simulink model "ControlledGrid"  (R2015b)
settings: configuration reference "ControlConfig" (kept outside this file)
InitFcn:
  | ControlInit();
undefined symbols (not defined in the file or in its folder): D1, Delta, Fnom, Grid_F, Grid_V, Rad2Deg, Ts
libraries: powerlib x16, powerlib_meascontrol x4, simulink x1
settings Model: Creator=Emilio  LastModifiedBy=Emilio
settings ConfigSetRef: SourceLocation=Base Workspace

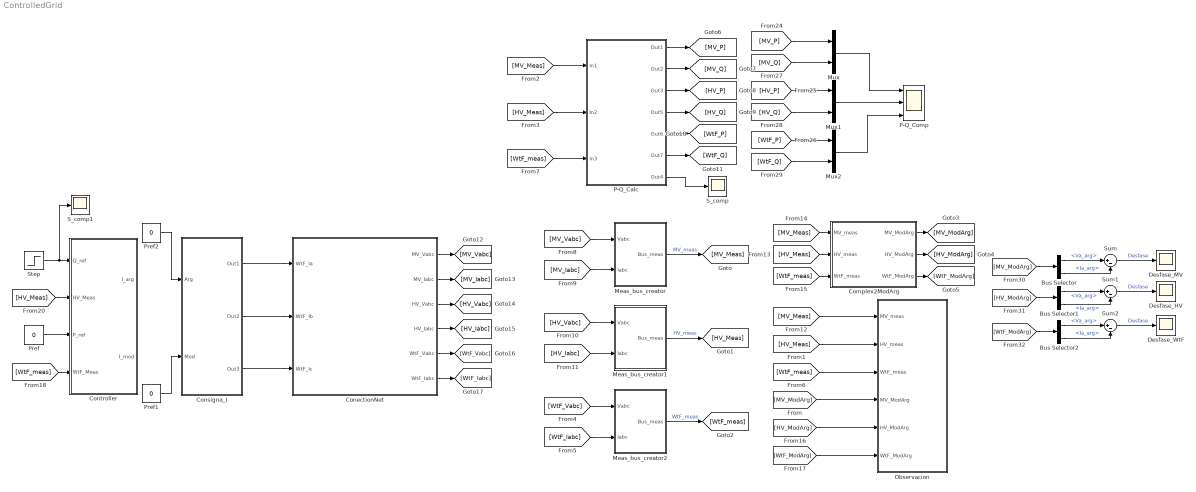
== system ControlledGrid ==
  Bus Selector : BusSelector  OutputSignals=V_ModArg.Va_arg,I_ModArg.Ia_arg
  Bus Selector1 : BusSelector  OutputSignals=V_ModArg.Va_arg,I_ModArg.Ia_arg
  Bus Selector2 : BusSelector  OutputSignals=V_ModArg.Va_arg,I_ModArg.Ia_arg
  Complex2ModArg : Subsystem
  ConectionNet : Subsystem
  Consigna_I : Subsystem
  Controller : Subsystem
  Desfase_HV : Scope
  Desfase_MV : Scope
  Desfase_WtF : Scope
  Meas_bus_creator : Subsystem
  Meas_bus_creator1 : Subsystem
  Meas_bus_creator2 : Subsystem
  Mux : Mux  Inputs=2
  Mux1 : Mux  Inputs=2
  Mux2 : Mux  Inputs=2
  Observacion : Subsystem
  P-Q_Calc : Subsystem
  P-Q_Comp : Scope  NumInputPorts=3
  Pref : Constant  Value=0
  Pref1 : Constant  Value=0
  Pref2 : Constant  Value=0
  S_comp : Scope
  S_comp1 : Scope
  Step : Step  After=4e6  SampleTime=0
  Sum : Sum  Inputs=|+-
  Sum1 : Sum  Inputs=|+-
  Sum2 : Sum  Inputs=|+-
  wires:
  [MV_Meas] -> P-Q_Calc/1(In1)
  [HV_Meas] -> P-Q_Calc/2(In2)
  P-Q_Calc/7(Out4) -> S_comp/1
  [MV_Vabc] -> Meas_bus_creator/1(Vabc)
  [MV_Iabc] -> Meas_bus_creator/2(Iabc)
  Meas_bus_creator/1(Bus_meas) -> [MV_Meas]  "MV_meas"
  [HV_Vabc] -> Meas_bus_creator1/1(Vabc)
  [HV_Iabc] -> Meas_bus_creator1/2(Iabc)
  Meas_bus_creator1/1(Bus_meas) -> [HV_Meas]  "HV_meas"
  [WtF_Vabc] -> Meas_bus_creator2/1(Vabc)
  [WtF_Iabc] -> Meas_bus_creator2/2(Iabc)
  Meas_bus_creator2/1(Bus_meas) -> [WtF_meas]  "WtF_meas"
  [WtF_meas] -> P-Q_Calc/3(In3)
  [MV_Meas] -> Observacion/1(MV_meas)
  [HV_Meas] -> Observacion/2(HV_meas)
  [WtF_meas] -> Observacion/3(WtF_meas)
  [MV_ModArg] -> Observacion/4(MV_ModArg)
  [HV_ModArg] -> Observacion/5(HV_ModArg)
  [WtF_ModArg] -> Observacion/6(WtF_ModArg)
  P-Q_Calc/1(Out1) -> [MV_P]
  P-Q_Calc/2(Out2) -> [MV_Q]
  P-Q_Calc/3(Out3) -> [HV_P]
  P-Q_Calc/4(Out5) -> [HV_Q]
  P-Q_Calc/5(Out6) -> [WtF_P]
  P-Q_Calc/6(Out7) -> [WtF_Q]
  ConectionNet/1(MV_Vabc) -> [MV_Vabc]
  ConectionNet/2(MV_Iabc) -> [MV_Iabc]
  ConectionNet/3(HV_Vabc) -> [HV_Vabc]
  ConectionNet/4(HV_Iabc) -> [HV_Iabc]
  ConectionNet/5(WtF_Vabc) -> [WtF_Vabc]
  ConectionNet/6(WtF_Iabc) -> [WtF_Iabc]
  [MV_Meas] -> Complex2ModArg/1(MV_meas)
  [HV_Meas] -> Complex2ModArg/2(HV_meas)
  [WtF_meas] -> Complex2ModArg/3(WtF_meas)
  Complex2ModArg/1(MV_ModArg) -> [MV_ModArg]
  Complex2ModArg/2(HV_ModArg) -> [HV_ModArg]
  Complex2ModArg/3(WtF_ModArg) -> [WtF_ModArg]
  [MV_P] -> Mux/1
  [MV_Q] -> Mux/2
  [HV_Q] -> Mux1/2
  [HV_P] -> Mux1/1
  [WtF_P] -> Mux2/1
  [WtF_Q] -> Mux2/2
  Mux/1 -> P-Q_Comp/1
  Mux1/1 -> P-Q_Comp/2
  Mux2/1 -> P-Q_Comp/3
  [MV_ModArg] -> Bus Selector/1
  Bus Selector/1 -> Sum/1  "<Va_arg>"
  Bus Selector/2 -> Sum/2  "<Ia_arg>"
  Sum/1 -> Desfase_MV/1  "Desfase"
  [HV_ModArg] -> Bus Selector1/1
  Bus Selector1/1 -> Sum1/1  "<Va_arg>"
  Bus Selector1/2 -> Sum1/2  "<Ia_arg>"
  Sum1/1 -> Desfase_HV/1  "Desfase"
  Bus Selector2/1 -> Sum2/1  "<Va_arg>"
  Bus Selector2/2 -> Sum2/2  "<Ia_arg>"
  Sum2/1 -> Desfase_WtF/1  "Desfase"
  [WtF_ModArg] -> Bus Selector2/1
  Step/1 -> S_comp1/1, Controller/1(Q_ref)
  [HV_Meas] -> Controller/2(HV_Meas)
  Pref/1 -> Controller/3(P_ref)
  [WtF_meas] -> Controller/4(WtF_Meas)
  Consigna_I/1(Out1) -> ConectionNet/1(WtF_Ia)
  Consigna_I/2(Out2) -> ConectionNet/2(WtF_Ib)
  Consigna_I/3(Out3) -> ConectionNet/3(WtF_Ic)
  Pref1/1 -> Consigna_I/2(Mod)
  Pref2/1 -> Consigna_I/1(Arg)

== system ControlledGrid/Complex2ModArg ==
  MV_meas : Inport
  HV_meas : Inport  Port=2
  WtF_meas : Inport  Port=3
  Bus Creator1 : BusCreator  Inputs=2
  Bus Creator2 : BusCreator  Inputs=2
  Bus Creator3 : BusCreator  Inputs=2
  Bus Selector3 : BusSelector  OutputSignals=V_meas.Va,V_meas.Vb,V_meas.Vc,I_meas.Ia,I_meas.Ib,I_meas.Ic
  Bus Selector4 : BusSelector  OutputSignals=V_meas.Va,V_meas.Vb,V_meas.Vc,I_meas.Ia,I_meas.Ib,I_meas.Ic
  Bus Selector5 : BusSelector  OutputSignals=V_meas.Va,V_meas.Vb,V_meas.Vc,I_meas.Ia,I_meas.Ib,I_meas.Ic
  HV_mod&arg : Subsystem
  MV_mod&arg : Subsystem
  WtF_mod&arg : Subsystem
  MV_ModArg : Outport
  HV_ModArg : Outport  Port=2
  WtF_ModArg : Outport  Port=3
  wires:
  Bus Selector4/1 -> WtF_mod&arg/1(In1)  "<Va>"
  Bus Selector3/1 -> HV_mod&arg/1(In1)  "<Va>"
  Bus Selector3/2 -> HV_mod&arg/2(In2)  "<Vb>"
  Bus Selector3/3 -> HV_mod&arg/3(In3)  "<Vc>"
  Bus Selector3/4 -> HV_mod&arg/4(In4)  "<Ia>"
  Bus Selector3/6 -> HV_mod&arg/6(In6)  "<Ic>"
  HV_mod&arg/1(Out1) -> Bus Creator3/1
  HV_meas/1 -> Bus Selector3/1
  HV_mod&arg/2(Out2) -> Bus Creator3/2
  WtF_meas/1 -> Bus Selector4/1
  Bus Selector3/5 -> HV_mod&arg/5(In5)  "<Ib>"
  Bus Selector4/6 -> WtF_mod&arg/6(In6)  "<Ic>"
  MV_mod&arg/1(Out1) -> Bus Creator2/1
  Bus Selector5/3 -> MV_mod&arg/3(In3)  "<Vc>"
  Bus Selector4/3 -> WtF_mod&arg/3(In3)  "<Vc>"
  Bus Selector4/2 -> WtF_mod&arg/2(In2)  "<Vb>"
  Bus Selector4/5 -> WtF_mod&arg/5(In5)  "<Ib>"
  Bus Creator3/1 -> HV_ModArg/1  "HV_ModArg"
  Bus Selector5/1 -> MV_mod&arg/1(In1)  "<Va>"
  Bus Selector5/6 -> MV_mod&arg/6(In6)  "<Ic>"
  Bus Selector5/5 -> MV_mod&arg/5(In5)  "<Ib>"
  Bus Creator2/1 -> MV_ModArg/1  "MV_ModArg"
  Bus Selector5/2 -> MV_mod&arg/2(In2)  "<Vb>"
  Bus Creator1/1 -> WtF_ModArg/1  "WtF_ModArg"
  WtF_mod&arg/1(Out1) -> Bus Creator1/1
  WtF_mod&arg/2(Out2) -> Bus Creator1/2
  MV_mod&arg/2(Out2) -> Bus Creator2/2
  Bus Selector4/4 -> WtF_mod&arg/4(In4)  "<Ia>"
  Bus Selector5/4 -> MV_mod&arg/4(In4)  "<Ia>"
  MV_meas/1 -> Bus Selector5/1

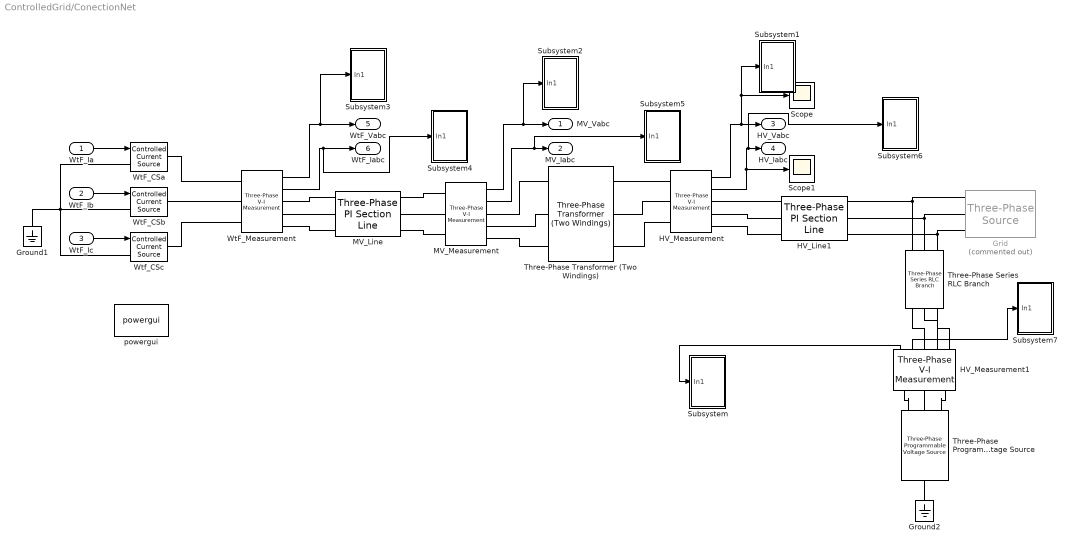
== system ControlledGrid/ConectionNet ==
  WtF_Ia : Inport
  WtF_Ib : Inport  Port=2
  WtF_Ic : Inport  Port=3
  Grid : powerlib/Electrical Sources/Three-Phase Source  Commented=on  InternalConnection=Yg  VoltagePhases=off  Voltage=Grid_V  PhaseAngle=0  Voltage_phases=[25e3 25e3 25e3]/sqrt(3)  PhaseAngles_phases=[0 -120 +120]  Frequency=Grid_F  NonIdealSource=on  SpecifyImpedance=on  Resistance=0.8929  Inductance=16.58e-3  ShortCircuitLevel=100e6  BaseVoltage=25e3  XRratio=7  BusType=PQ  Pref=10e3  Qref=0  Prefabc=[10e3, 10e3, 10e3]  Qrefabc=[0, 0, 0]  Qmin=-inf  Qmax=inf
  Ground1 : powerlib/Elements/Ground  LConnTagsString=a
  Ground2 : powerlib/Elements/Ground  LConnTagsString=a
  HV_Line1 : powerlib/Elements/Three-Phase PI Section Line  LConnTagsString=a|b|c  RConnTagsString=A|B|C  Frequency=Fnom  Resistances=[ 0.01273 0.3864]  Inductances="[ 0.9337e-3  4.1264e-3]"  Capacitances=[0.16e-6 0.16e-6]  Length=100
  HV_Measurement : powerlib/Measurements/Three-Phase V-I Measurement  VoltageMeasurement=phase-to-ground  SetLabelV=off  LabelV=HV_Vabc  Vpu=off  VpuLL=off  CurrentMeasurement=yes  SetLabelI=off  LabelI=HV_Iabc  Ipu=off  Pbase=100e6  Vbase=500e3  OutputType=Complex  PhasorSimulation=on  PSBequivalent=0
  HV_Measurement1 : powerlib/Measurements/Three-Phase V-I Measurement  VoltageMeasurement=phase-to-ground  SetLabelV=off  LabelV=HV_Vabc  Vpu=off  VpuLL=off  CurrentMeasurement=yes  SetLabelI=off  LabelI=HV_Iabc  Ipu=off  Pbase=100e6  Vbase=500e3  OutputType=Complex  PhasorSimulation=on  PSBequivalent=0
  MV_Line : powerlib/Elements/Three-Phase PI Section Line  LConnTagsString=a|b|c  RConnTagsString=A|B|C  Frequency=50  Resistances=[ 0.01273 0.3864]  Inductances="[ 0.9337e-3  4.1264e-3]"  Capacitances="[ 0.16e-6  0.16e-6]"  Length=20
  MV_Measurement : powerlib/Measurements/Three-Phase V-I Measurement  VoltageMeasurement=phase-to-ground  SetLabelV=off  LabelV=MV_Vabc  Vpu=off  VpuLL=off  CurrentMeasurement=yes  SetLabelI=off  LabelI=MV_Iabc  Ipu=off  Pbase=100e6  Vbase=500e3  OutputType=Complex  PhasorSimulation=on  PSBequivalent=0
  Scope : Scope
  Scope1 : Scope
  Subsystem : Subsystem
  Subsystem1 : Subsystem
  Subsystem2 : Subsystem
  Subsystem3 : Subsystem
  Subsystem4 : Subsystem
  Subsystem5 : Subsystem
  Subsystem6 : Subsystem
  Subsystem7 : Subsystem
  Three-Phase Programmable Voltage Source : powerlib/Electrical Sources/Three-Phase Programmable Voltage Source  PositiveSequence="[Grid_V  0 Fnom]"  VariationEntity=Amplitude  VariationType=Modulation  VariationTypeAlt=Step  VariationStep=0.5  VariationRate=10  VariationMagnitude=0  VariationFrequency=0.10  VariationTiming=[0 10]  VariationPhaseA=off  Amplitudes=[1 0.8 1.2 1.0]  TimeValues=[0 0.1 0.15 0.2]  HarmonicGeneration=off  HarmonicA=[3 0.2 -25 0]  HarmonicB=[2 0.15 35 2]  Timing="[0.05  3]"  BusType=PQ  Pref=0  Qref=0  Qmin=-inf  Qmax=inf
  Three-Phase Series RLC Branch : powerlib/Elements/Three-Phase Series RLC Branch  LConnTagsString=A|B|C  RConnTagsString=A|B|C  BranchType=RL  Resistance=1  Inductance=7  Capacitance=0  Measurements=None
  Three-Phase Transformer (Two Windings) : powerlib/Elements/Three-Phase Transformer (Two Windings)  Winding1Connection=Delta (D1)  Winding2Connection=Delta (D1)  CoreType=Three single-phase transformers  SetSaturation=off  Hysteresis=off  DataFile='hysteresis'  SetInitialFlux=off  Measurements=None  UNITS=SI  NominalPower=[ 100e3 , 50 ]  Winding1=[22000 9.68 0.030812]  Winding2=[4e+05 3200 10.186]  Rm=2.42e+06  Lm=7703.1  L0=7.7033  Saturation=[0 0;0.0089072 68.613;3.7113 86.91]  InitialFluxes=[45.742 -45.742 40.024]  MoreParameters=off  BreakLoop=off  DataType=on  TransfoNumber=1
  WtF_CSa : powerlib/Electrical Sources/Controlled Current Source  Initialize=on  Source_Type=AC  Amplitude=0  Phase=0  Frequency=Fnom  Measurements=None
  WtF_CSb : powerlib/Electrical Sources/Controlled Current Source  Initialize=on  Source_Type=AC  Amplitude=0  Phase=120  Frequency=Fnom  Measurements=None
  WtF_Measurement : powerlib/Measurements/Three-Phase V-I Measurement  VoltageMeasurement=phase-to-ground  SetLabelV=off  LabelV=WtF_Vabc  Vpu=off  VpuLL=off  CurrentMeasurement=yes  SetLabelI=off  LabelI=WtF_Iabc  Ipu=off  Pbase=100e6  Vbase=500e3  OutputType=Complex  PhasorSimulation=on  PSBequivalent=0
  Wtf_CSc : powerlib/Electrical Sources/Controlled Current Source  Initialize=on  Source_Type=AC  Amplitude=0  Phase=-120  Frequency=Fnom  Measurements=None
  powergui : powerlib/powergui  Priority=1  SimulationMode=Phasor  SolverType=Tustin/Backward Euler (TBE)  SampleTime=50e-6  frequency=Fnom  SPID=off  DisableSnubberDevices=off  DisableRonSwitches=off  DisableVfSwitches=off  SwTol=0  DisplayEquations=off  Interpol=off  ExternalGateDelay=off  methode=off  Ts=10  FunctionMessages=off  echomessages=off  HookPort=off  EnableUseOfTLC=off  x0status=blocks  frequencyindice=50  Pbase=100e6  ErrMax=1e-4  Iterations=50  UnitsV=V  UnitsW=W  buscounter=0  RestoreLinks=warning  ResistiveCurrentMeasurement=off  Frange=[0:2:500]  Ylog=off  Xlog=on  ShowGrid=off  save=off  variable=ZData  structure=0  ZoomFFT=off  StartTime=0.0  cycles=1  DisplayStyle=1  fundamental=60  FreqAxis=off  MaxFrequency=1000  frequencyindicesteady=1  RmsSteady=1  display=off
  MV_Vabc : Outport
  MV_Iabc : Outport  Port=2
  HV_Vabc : Outport  Port=3
  HV_Iabc : Outport  Port=4
  WtF_Vabc : Outport  Port=5
  WtF_Iabc : Outport  Port=6
  wires:
  WtF_Ia/1 -> WtF_CSa/1
  WtF_Ib/1 -> WtF_CSb/1
  WtF_Ic/1 -> Wtf_CSc/1
  MV_Measurement/1 -> Subsystem2/1(In1), MV_Vabc/1
  HV_Measurement/1 -> Subsystem1/1(In1), Scope/1, HV_Vabc/1
  HV_Measurement/2 -> Subsystem6/1(In1), HV_Iabc/1, Scope1/1
  MV_Measurement/2 -> Subsystem5/1(In1), MV_Iabc/1
  WtF_Measurement/1 -> Subsystem3/1(In1), WtF_Vabc/1
  WtF_Measurement/2 -> WtF_Iabc/1, Subsystem4/1(In1)
  HV_Measurement1/2 -> Subsystem7/1(In1)
  HV_Measurement1/1 -> Subsystem/1(In1)
  connections:
  HV_Measurement/LConn2 -- Three-Phase Transformer (Two Windings)/RConn2
  Three-Phase Series RLC Branch/LConn3 -- HV_Line1/RConn3 -- Grid/RConn1
  Three-Phase Series RLC Branch/LConn1 -- Grid/RConn3 -- HV_Line1/RConn1
  Three-Phase Series RLC Branch/LConn2 -- HV_Line1/RConn2 -- Grid/RConn2
  HV_Measurement/LConn1 -- Three-Phase Transformer (Two Windings)/RConn1
  HV_Measurement/LConn3 -- Three-Phase Transformer (Two Windings)/RConn3
  MV_Measurement/RConn2 -- Three-Phase Transformer (Two Windings)/LConn2
  MV_Measurement/RConn3 -- Three-Phase Transformer (Two Windings)/LConn3
  MV_Measurement/RConn1 -- Three-Phase Transformer (Two Windings)/LConn1
  MV_Line/RConn1 -- MV_Measurement/LConn1
  MV_Line/RConn3 -- MV_Measurement/LConn3
  WtF_Measurement/LConn3 -- Wtf_CSc/RConn1
  WtF_Measurement/LConn1 -- WtF_CSa/RConn1
  MV_Line/RConn2 -- MV_Measurement/LConn2
  WtF_Measurement/LConn2 -- WtF_CSb/RConn1
  WtF_Measurement/RConn3 -- MV_Line/LConn3
  WtF_Measurement/RConn2 -- MV_Line/LConn2
  WtF_Measurement/RConn1 -- MV_Line/LConn1
  Wtf_CSc/LConn1 -- Ground1/LConn1 -- WtF_CSb/LConn1 -- WtF_CSa/LConn1
  Three-Phase Programmable Voltage Source/RConn1 -- HV_Measurement1/LConn1
  Three-Phase Programmable Voltage Source/RConn2 -- HV_Measurement1/LConn2
  Three-Phase Programmable Voltage Source/RConn3 -- HV_Measurement1/LConn3
  HV_Measurement1/RConn1 -- Three-Phase Series RLC Branch/RConn1
  HV_Measurement1/RConn2 -- Three-Phase Series RLC Branch/RConn2
  HV_Measurement1/RConn3 -- Three-Phase Series RLC Branch/RConn3
  Ground2/LConn1 -- Three-Phase Programmable Voltage Source/LConn1
  HV_Line1/LConn1 -- HV_Measurement/RConn1
  HV_Measurement/RConn2 -- HV_Line1/LConn2
  HV_Measurement/RConn3 -- HV_Line1/LConn3

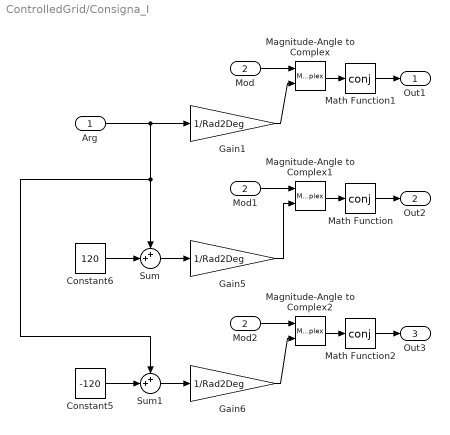
== system ControlledGrid/Consigna_I ==
  Arg : Inport
  Mod : Inport  Port=2
  Constant5 : Constant  Value=-120
  Constant6 : Constant  Value=120
  Gain1 : Gain  Gain=1/Rad2Deg
  Gain5 : Gain  Gain=1/Rad2Deg
  Gain6 : Gain  Gain=1/Rad2Deg
  Magnitude-Angle to Complex : MagnitudeAngleToComplex
  Magnitude-Angle to Complex1 : MagnitudeAngleToComplex
  Magnitude-Angle to Complex2 : MagnitudeAngleToComplex
  Math Function : Math  Operator=conj  SaturateOnIntegerOverflow=on
  Math Function1 : Math  Operator=conj  SaturateOnIntegerOverflow=on
  Math Function2 : Math  Operator=conj  SaturateOnIntegerOverflow=on
  Mod1 : InportShadow  Port=2
  Mod2 : InportShadow  Port=2
  Sum : Sum  Inputs=++|
  Sum1 : Sum  Inputs=++|
  Out1 : Outport
  Out2 : Outport  Port=2
  Out3 : Outport  Port=3
  wires:
  Gain1/1 -> Magnitude-Angle to Complex/2
  Constant6/1 -> Sum/2
  Sum/1 -> Gain5/1
  Constant5/1 -> Sum1/2
  Sum1/1 -> Gain6/1
  Arg/1 -> Sum1/1, Sum/1, Gain1/1
  Mod/1 -> Magnitude-Angle to Complex/1
  Mod1/1 -> Magnitude-Angle to Complex1/1
  Mod2/1 -> Magnitude-Angle to Complex2/1
  Gain6/1 -> Magnitude-Angle to Complex2/2
  Gain5/1 -> Magnitude-Angle to Complex1/2
  Magnitude-Angle to Complex2/1 -> Math Function2/1
  Magnitude-Angle to Complex1/1 -> Math Function/1
  Magnitude-Angle to Complex/1 -> Math Function1/1
  Math Function/1 -> Out2/1
  Math Function1/1 -> Out1/1
  Math Function2/1 -> Out3/1

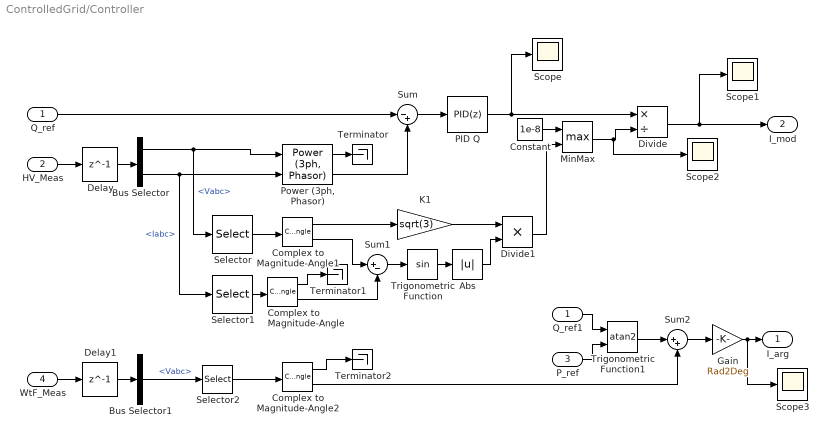
== system ControlledGrid/Controller ==
  Q_ref : Inport
  HV_Meas : Inport  Port=2  OutDataTypeStr=Bus: HV_meas
  P_ref : Inport  Port=3
  WtF_Meas : Inport  Port=4  OutDataTypeStr=Bus: WtF_meas
  Abs : Abs
  Bus Selector : BusSelector  OutputSignals=V_meas.Vabc,I_meas.Iabc
  Bus Selector1 : BusSelector  OutputSignals=V_meas.Vabc
  Complex to Magnitude-Angle : ComplexToMagnitudeAngle
  Complex to Magnitude-Angle1 : ComplexToMagnitudeAngle
  Complex to Magnitude-Angle2 : ComplexToMagnitudeAngle
  Constant : Constant  Value=1e-8
  Delay : Delay  DelayLength=1  InitialCondition=0  SampleTime=Ts
  Delay1 : Delay  DelayLength=1  InitialCondition=0  SampleTime=Ts
  Divide : Product  Inputs=*/
  Divide1 : Product  Inputs=**
  Gain : Gain  Gain=Rad2Deg
  K1 : Gain  Gain=sqrt(3)  SaturateOnIntegerOverflow=on  OutDataTypeStr=Inherit: Same as input  ParamDataTypeStr=Inherit: Same as input
  MinMax : MinMax  Function=max  Inputs=2
  PID Q : simulink/Continuous/PID Controller  Controller=PID  TimeDomain=Discrete-time  SampleTime=Ts  IntegratorMethod=Forward Euler  FilterMethod=Forward Euler  Form=Parallel  UseFilter=on  ControllerParametersSource=internal  P=1.25  I=0  D=0  N=100  InitialConditionSource=internal  InitialConditionForIntegrator=0  InitialConditionForFilter=0  ExternalReset=none  LimitOutput=off  UpperSaturationLimit=inf  LowerSaturationLimit=-inf  LinearizeAsGain=off  AntiWindupMode=none  Kb=1  TrackingMode=off  Kt=1  PParamMin=[]  PParamMax=[]  IParamMin=[]  IParamMax=[]  DParamMin=[]  DParamMax=[]  NParamMin=[]  NParamMax=[]  KbParamMin=[]  KbParamMax=[]  KtParamMin=[]  KtParamMax=[]  POutMin=[]  POutMax=[]  IOutMin=[]  IOutMax=[]  DOutMin=[]  DOutMax=[]  NOutMin=[]  NOutMax=[]  KbOutMin=[]  KbOutMax=[]  KtOutMin=[]  KtOutMax=[]  IntegratorOutMin=[]  IntegratorOutMax=[]  FilterOutMin=[]  FilterOutMax=[]  SumOutMin=[]  SumOutMax=[]  SumI1OutMin=[]  SumI1OutMax=[]  SumI2OutMin=[]  SumI2OutMax=[]  SumI3OutMin=[]  SumI3OutMax=[]  SumDOutMin=[]  SumDOutMax=[]  SaturationOutMin=[]  SaturationOutMax=[]  IntegratorContinuousStateAttributes=''  IntegratorStateMustResolveToSignalObject=off  IntegratorRTWStateStorageClass=Auto  FilterContinuousStateAttributes=''  FilterStateMustResolveToSignalObject=off  FilterRTWStateStorageClass=Auto  DifferentiatorICPrevScaledInput=0  DifferentiatorOutMin=[]  DifferentiatorOutMax=[]
  "Power (3ph, Phasor)" : powerlib_meascontrol/Measurements/Power (3ph, Phasor)
  Q_ref1 : InportShadow
  Scope{,1..3} (4 alike) : Scope
  Selector : Selector  InputPortWidth=3  IndexOptions=Index vector (dialog)  Indices=[1 ]  OutputSizes=1
  Selector1 : Selector  InputPortWidth=3  IndexOptions=Index vector (dialog)  Indices=[1 ]  OutputSizes=1
  Selector2 : Selector  InputPortWidth=3  IndexOptions=Index vector (dialog)  Indices=[1 ]  OutputSizes=1
  Sum : Sum  Inputs=|-+
  Sum1 : Sum  Inputs=|+-
  Sum2 : Sum  Inputs=|++
  Terminator : Terminator
  Terminator1 : Terminator
  Terminator2 : Terminator
  Trigonometric Function : Trigonometry
  Trigonometric Function1 : Trigonometry  Operator=atan2
  I_arg : Outport
  I_mod : Outport  Port=2
  wires:
  HV_Meas/1 -> Delay/1
  Bus Selector/1 -> "Power (3ph, Phasor)"/1, Selector/1  "<Vabc>"
  Bus Selector/2 -> "Power (3ph, Phasor)"/2, Selector1/1  "<Iabc>"
  Divide/1 -> Scope1/1, I_mod/1
  Delay/1 -> Bus Selector/1
  PID Q/1 -> Scope/1, Divide/1
  Sum/1 -> PID Q/1
  Q_ref/1 -> Sum/1
  Complex to Magnitude-Angle1/2 -> Sum1/1
  Complex to Magnitude-Angle/2 -> Sum1/2
  Sum1/1 -> Trigonometric Function/1
  Trigonometric Function/1 -> Abs/1
  K1/1 -> Divide1/1
  Complex to Magnitude-Angle1/1 -> K1/1
  "Power (3ph, Phasor)"/1 -> Terminator/1
  Selector/1 -> Complex to Magnitude-Angle1/1
  Selector1/1 -> Complex to Magnitude-Angle/1
  WtF_Meas/1 -> Delay1/1
  Delay1/1 -> Bus Selector1/1
  Bus Selector1/1 -> Selector2/1  "<Vabc>"
  Selector2/1 -> Complex to Magnitude-Angle2/1
  Sum2/1 -> Gain/1
  Complex to Magnitude-Angle2/2 -> Sum2/2
  Complex to Magnitude-Angle/1 -> Terminator1/1
  Complex to Magnitude-Angle2/1 -> Terminator2/1
  "Power (3ph, Phasor)"/2 -> Sum/2
  Trigonometric Function1/1 -> Sum2/1
  P_ref/1 -> Trigonometric Function1/2
  Q_ref1/1 -> Trigonometric Function1/1
  MinMax/1 -> Scope2/1, Divide/2
  Divide1/1 -> MinMax/2
  Constant/1 -> MinMax/1
  Abs/1 -> Divide1/2
  Gain/1 -> Scope3/1, I_arg/1

== system ControlledGrid/Meas_bus_creator ==
  note: Creacion de los buses de medidas de los parametros de la red
  Vabc : Inport
  Iabc : Inport  Port=2
  " " : ComplexToRealImag
  "  " : ComplexToRealImag
  Bus Creator : BusCreator  Inputs=2
  Bus Creator1 : BusCreator  Inputs=6
  Bus Creator2 : BusCreator  Inputs=6
  Demux4 : Demux  Outputs=3
  Demux5 : Demux  Outputs=3
  Bus_meas : Outport  OutDataTypeStr=Bus: MV_meas
  wires:
  Demux4/3 -> Bus Creator1/6  "Vc"
  Bus Creator1/1 -> Bus Creator/1  "V_meas"
  Bus Creator2/1 -> Bus Creator/2  "I_meas"
  Demux5/1 -> " "/1, Bus Creator2/2  "Ia"
  "  "/1 -> Bus Creator1/3  "Va_real"
  Bus Creator/1 -> Bus_meas/1
  Demux5/2 -> Bus Creator2/5  "Ib"
  " "/2 -> Bus Creator2/4  "Ia_img"
  Demux5/3 -> Bus Creator2/6  "Ic"
  Demux4/2 -> Bus Creator1/5  "Vb"
  Demux4/1 -> Bus Creator1/2, "  "/1  "Va"
  "  "/2 -> Bus Creator1/4  "Va_img"
  Iabc/1 -> Bus Creator2/1, Demux5/1  "Iabc"
  Vabc/1 -> Bus Creator1/1, Demux4/1  "Vabc"
  " "/1 -> Bus Creator2/3  "Ia_real"

== system ControlledGrid/Meas_bus_creator1 ==
  note: Creacion de los buses de medidas de los parametros de la red
  Vabc : Inport
  Iabc : Inport  Port=2
  " " : ComplexToRealImag
  "  " : ComplexToRealImag
  Bus Creator : BusCreator  Inputs=2
  Bus Creator1 : BusCreator  Inputs=6
  Bus Creator2 : BusCreator  Inputs=6
  Demux4 : Demux  Outputs=3
  Demux5 : Demux  Outputs=3
  Bus_meas : Outport  OutDataTypeStr=Bus: MV_meas
  wires:
  " "/1 -> Bus Creator2/3  "Ia_real"
  Vabc/1 -> Demux4/1, Bus Creator1/1  "Vabc"
  Iabc/1 -> Demux5/1, Bus Creator2/1  "Iabc"
  "  "/2 -> Bus Creator1/4  "Va_img"
  Demux4/1 -> "  "/1, Bus Creator1/2  "Va"
  Demux4/2 -> Bus Creator1/5  "Vb"
  Demux5/3 -> Bus Creator2/6  "Ic"
  " "/2 -> Bus Creator2/4  "Ia_img"
  Demux5/2 -> Bus Creator2/5  "Ib"
  Bus Creator/1 -> Bus_meas/1
  "  "/1 -> Bus Creator1/3  "Va_real"
  Demux5/1 -> Bus Creator2/2, " "/1  "Ia"
  Bus Creator2/1 -> Bus Creator/2  "I_meas"
  Bus Creator1/1 -> Bus Creator/1  "V_meas"
  Demux4/3 -> Bus Creator1/6  "Vc"

== system ControlledGrid/Meas_bus_creator2 ==
  note: Creacion de los buses de medidas de los parametros de la red
  Vabc : Inport
  Iabc : Inport  Port=2
  " " : ComplexToRealImag
  "  " : ComplexToRealImag
  Bus Creator : BusCreator  Inputs=2
  Bus Creator1 : BusCreator  Inputs=6
  Bus Creator2 : BusCreator  Inputs=6
  Demux4 : Demux  Outputs=3
  Demux5 : Demux  Outputs=3
  Bus_meas : Outport  OutDataTypeStr=Bus: MV_meas
  wires:
  " "/1 -> Bus Creator2/3  "Ia_real"
  Vabc/1 -> Demux4/1, Bus Creator1/1  "Vabc"
  Iabc/1 -> Demux5/1, Bus Creator2/1  "Iabc"
  "  "/2 -> Bus Creator1/4  "Va_img"
  Demux4/1 -> "  "/1, Bus Creator1/2  "Va"
  Demux4/2 -> Bus Creator1/5  "Vb"
  Demux5/3 -> Bus Creator2/6  "Ic"
  " "/2 -> Bus Creator2/4  "Ia_img"
  Demux5/2 -> Bus Creator2/5  "Ib"
  Bus Creator/1 -> Bus_meas/1
  "  "/1 -> Bus Creator1/3  "Va_real"
  Demux5/1 -> Bus Creator2/2, " "/1  "Ia"
  Bus Creator2/1 -> Bus Creator/2  "I_meas"
  Bus Creator1/1 -> Bus Creator/1  "V_meas"
  Demux4/3 -> Bus Creator1/6  "Vc"

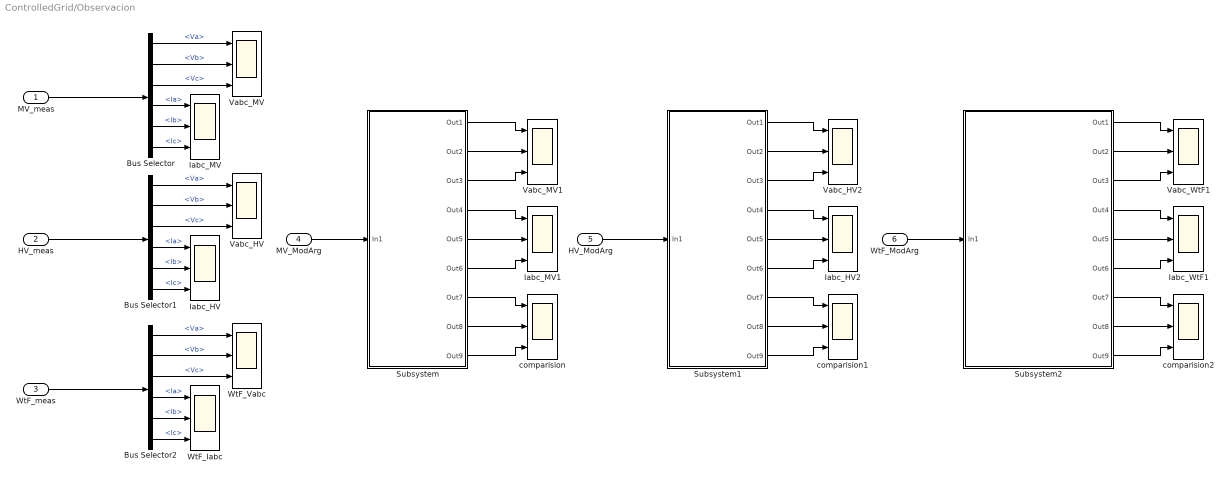
== system ControlledGrid/Observacion ==
  MV_meas : Inport  OutDataTypeStr=Bus: MV_meas
  HV_meas : Inport  Port=2  OutDataTypeStr=Bus: HV_meas
  WtF_meas : Inport  Port=3  OutDataTypeStr=Bus: WtF_meas
  MV_ModArg : Inport  Port=4  OutDataTypeStr=Bus: MV_ModArg
  HV_ModArg : Inport  Port=5  OutDataTypeStr=Bus: HV_ModArg
  WtF_ModArg : Inport  Port=6  OutDataTypeStr=Bus: WtF_ModArg
  Bus Selector : BusSelector  OutputSignals=V_meas.Va,V_meas.Vb,V_meas.Vc,I_meas.Ia,I_meas.Ib,I_meas.Ic
  Bus Selector1 : BusSelector  OutputSignals=V_meas.Va,V_meas.Vb,V_meas.Vc,I_meas.Ia,I_meas.Ib,I_meas.Ic
  Bus Selector2 : BusSelector  OutputSignals=V_meas.Va,V_meas.Vb,V_meas.Vc,I_meas.Ia,I_meas.Ib,I_meas.Ic
  Iabc_HV : Scope  NumInputPorts=3
  Iabc_HV2 : Scope  NumInputPorts=3
  Iabc_MV : Scope  NumInputPorts=3
  Iabc_MV1 : Scope  NumInputPorts=3
  Iabc_WtF1 : Scope  NumInputPorts=3
  Subsystem : Subsystem
  Subsystem1 : Subsystem
  Subsystem2 : Subsystem
  Vabc_HV : Scope  NumInputPorts=3
  Vabc_HV2 : Scope  NumInputPorts=3
  Vabc_MV : Scope  NumInputPorts=3
  Vabc_MV1 : Scope  NumInputPorts=3
  Vabc_WtF1 : Scope  NumInputPorts=3
  WtF_Iabc : Scope  NumInputPorts=3
  WtF_Vabc : Scope  NumInputPorts=3
  comparision : Scope  NumInputPorts=3
  comparision1 : Scope  NumInputPorts=3
  comparision2 : Scope  NumInputPorts=3
  wires:
  Bus Selector/6 -> Iabc_MV/3  "<Ic>"
  Bus Selector/3 -> Vabc_MV/3  "<Vc>"
  Bus Selector/1 -> Vabc_MV/1  "<Va>"
  Bus Selector/4 -> Iabc_MV/1  "<Ia>"
  Bus Selector/2 -> Vabc_MV/2  "<Vb>"
  Bus Selector/5 -> Iabc_MV/2  "<Ib>"
  Bus Selector1/1 -> Vabc_HV/1  "<Va>"
  Bus Selector1/4 -> Iabc_HV/1  "<Ia>"
  Bus Selector1/2 -> Vabc_HV/2  "<Vb>"
  Bus Selector2/1 -> WtF_Vabc/1  "<Va>"
  MV_meas/1 -> Bus Selector/1
  HV_meas/1 -> Bus Selector1/1
  Bus Selector2/2 -> WtF_Vabc/2  "<Vb>"
  Bus Selector1/6 -> Iabc_HV/3  "<Ic>"
  Bus Selector1/3 -> Vabc_HV/3  "<Vc>"
  WtF_meas/1 -> Bus Selector2/1
  Bus Selector1/5 -> Iabc_HV/2  "<Ib>"
  Bus Selector2/3 -> WtF_Vabc/3  "<Vc>"
  Bus Selector2/5 -> WtF_Iabc/2  "<Ib>"
  Bus Selector2/4 -> WtF_Iabc/1  "<Ia>"
  Bus Selector2/6 -> WtF_Iabc/3  "<Ic>"
  Subsystem1/1(Out1) -> Vabc_HV2/1
  Subsystem1/3(Out3) -> Vabc_HV2/3
  Subsystem1/5(Out5) -> Iabc_HV2/2
  Subsystem1/6(Out6) -> Iabc_HV2/3
  Subsystem1/8(Out8) -> comparision1/2
  Subsystem1/2(Out2) -> Vabc_HV2/2
  Subsystem1/7(Out7) -> comparision1/1
  Subsystem1/4(Out4) -> Iabc_HV2/1
  HV_ModArg/1 -> Subsystem1/1(In1)
  Subsystem1/9(Out9) -> comparision1/3
  Subsystem/9(Out9) -> comparision/3
  Subsystem/8(Out8) -> comparision/2
  MV_ModArg/1 -> Subsystem/1(In1)
  Subsystem/6(Out6) -> Iabc_MV1/3
  Subsystem/5(Out5) -> Iabc_MV1/2
  Subsystem/1(Out1) -> Vabc_MV1/1
  Subsystem/4(Out4) -> Iabc_MV1/1
  Subsystem/2(Out2) -> Vabc_MV1/2
  Subsystem/7(Out7) -> comparision/1
  Subsystem/3(Out3) -> Vabc_MV1/3
  WtF_ModArg/1 -> Subsystem2/1(In1)
  Subsystem2/2(Out2) -> Vabc_WtF1/2
  Subsystem2/3(Out3) -> Vabc_WtF1/3
  Subsystem2/1(Out1) -> Vabc_WtF1/1
  Subsystem2/4(Out4) -> Iabc_WtF1/1
  Subsystem2/5(Out5) -> Iabc_WtF1/2
  Subsystem2/6(Out6) -> Iabc_WtF1/3
  Subsystem2/7(Out7) -> comparision2/1
  Subsystem2/9(Out9) -> comparision2/3
  Subsystem2/8(Out8) -> comparision2/2

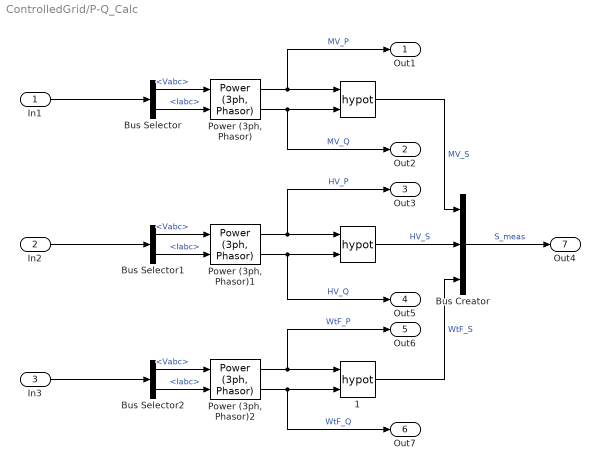
== system ControlledGrid/P-Q_Calc ==
  In1 : Inport  OutDataTypeStr=Bus: MV_meas
  In2 : Inport  Port=2  OutDataTypeStr=Bus: HV_meas
  In3 : Inport  Port=3  OutDataTypeStr=Bus: WtF_meas
  " " : Math  Operator=hypot  SaturateOnIntegerOverflow=on
  "  " : Math  Operator=hypot  SaturateOnIntegerOverflow=on
  "  1" : Math  Operator=hypot  SaturateOnIntegerOverflow=on
  Bus Creator : BusCreator  Inputs=3
  Bus Selector : BusSelector  OutputSignals=V_meas.Vabc,I_meas.Iabc
  Bus Selector1 : BusSelector  OutputSignals=V_meas.Vabc,I_meas.Iabc
  Bus Selector2 : BusSelector  OutputSignals=V_meas.Vabc,I_meas.Iabc
  "Power (3ph, Phasor)" : powerlib_meascontrol/Measurements/Power (3ph, Phasor)
  "Power (3ph, Phasor)1" : powerlib_meascontrol/Measurements/Power (3ph, Phasor)
  "Power (3ph, Phasor)2" : powerlib_meascontrol/Measurements/Power (3ph, Phasor)
  Out1 : Outport
  Out2 : Outport  Port=2
  Out3 : Outport  Port=3
  Out5 : Outport  Port=4
  Out6 : Outport  Port=5
  Out7 : Outport  Port=6
  Out4 : Outport  Port=7  OutDataTypeStr=Bus: S_meas
  wires:
  Bus Creator/1 -> Out4/1  "S_meas"
  "Power (3ph, Phasor)"/2 -> " "/2, Out2/1  "MV_Q"
  "Power (3ph, Phasor)1"/2 -> Out5/1, "  "/2  "HV_Q"
  " "/1 -> Bus Creator/1  "MV_S"
  "Power (3ph, Phasor)1"/1 -> Out3/1, "  "/1  "HV_P"
  "  "/1 -> Bus Creator/2  "HV_S"
  "Power (3ph, Phasor)"/1 -> " "/1, Out1/1  "MV_P"
  In1/1 -> Bus Selector/1
  Bus Selector/1 -> "Power (3ph, Phasor)"/1  "<Vabc>"
  Bus Selector/2 -> "Power (3ph, Phasor)"/2  "<Iabc>"
  In2/1 -> Bus Selector1/1
  Bus Selector1/1 -> "Power (3ph, Phasor)1"/1  "<Vabc>"
  Bus Selector1/2 -> "Power (3ph, Phasor)1"/2  "<Iabc>"
  "Power (3ph, Phasor)2"/2 -> "  1"/2, Out7/1  "WtF_Q"
  "Power (3ph, Phasor)2"/1 -> "  1"/1, Out6/1  "WtF_P"
  "  1"/1 -> Bus Creator/3  "WtF_S"
  In3/1 -> Bus Selector2/1
  Bus Selector2/1 -> "Power (3ph, Phasor)2"/1  "<Vabc>"
  Bus Selector2/2 -> "Power (3ph, Phasor)2"/2  "<Iabc>"

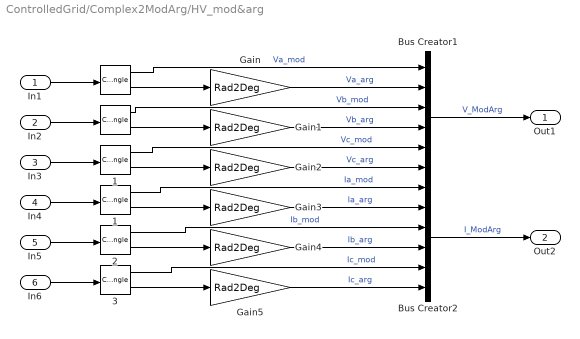
== system ControlledGrid/Complex2ModArg/HV_mod&arg ==
  In1 : Inport
  In2 : Inport  Port=2
  In3 : Inport  Port=3
  In4 : Inport  Port=4
  In5 : Inport  Port=5
  In6 : Inport  Port=6
  " " : ComplexToMagnitudeAngle
    {,1..3} (4 alike) : ComplexToMagnitudeAngle
  " 1" : ComplexToMagnitudeAngle
  Bus Creator1 : BusCreator  Inputs=6
  Bus Creator2 : BusCreator  Inputs=6
  Gain{,1..5} (6 alike) : Gain  Gain=Rad2Deg
  Out1 : Outport  OutDataTypeStr=Bus: V_ModArg
  Out2 : Outport  Port=2  OutDataTypeStr=Bus: I_ModArg
  wires:
  " "/2 -> Gain/1
  "  3"/2 -> Gain5/1
  " 1"/2 -> Gain3/1
  "  2"/1 -> Bus Creator2/3  "Ib_mod"
  " 1"/1 -> Bus Creator2/1  "Ia_mod"
  Gain2/1 -> Bus Creator1/6  "Vc_arg"
  "  1"/2 -> Gain2/1
  Gain1/1 -> Bus Creator1/4  "Vb_arg"
  Bus Creator1/1 -> Out1/1  "V_ModArg"
  "  "/2 -> Gain1/1
  "  "/1 -> Bus Creator1/3  "Vb_mod"
  "  2"/2 -> Gain4/1
  Gain/1 -> Bus Creator1/2  "Va_arg"
  Gain5/1 -> Bus Creator2/6  "Ic_arg"
  " "/1 -> Bus Creator1/1  "Va_mod"
  "  1"/1 -> Bus Creator1/5  "Vc_mod"
  Gain3/1 -> Bus Creator2/2  "Ia_arg"
  Bus Creator2/1 -> Out2/1  "I_ModArg"
  Gain4/1 -> Bus Creator2/4  "Ib_arg"
  "  3"/1 -> Bus Creator2/5  "Ic_mod"
  In5/1 -> "  2"/1
  In6/1 -> "  3"/1
  In4/1 -> " 1"/1
  In3/1 -> "  1"/1
  In2/1 -> "  "/1
  In1/1 -> " "/1

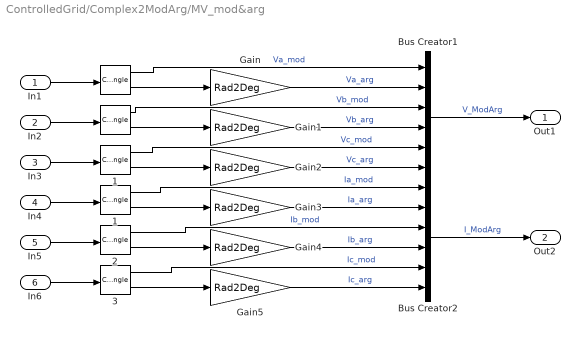
== system ControlledGrid/Complex2ModArg/MV_mod&arg ==
  In1 : Inport
  In2 : Inport  Port=2
  In3 : Inport  Port=3
  In4 : Inport  Port=4
  In5 : Inport  Port=5
  In6 : Inport  Port=6
  " " : ComplexToMagnitudeAngle
    {,1..3} (4 alike) : ComplexToMagnitudeAngle
  " 1" : ComplexToMagnitudeAngle
  Bus Creator1 : BusCreator  Inputs=6
  Bus Creator2 : BusCreator  Inputs=6
  Gain{,1..5} (6 alike) : Gain  Gain=Rad2Deg
  Out1 : Outport  OutDataTypeStr=Bus: V_ModArg
  Out2 : Outport  Port=2  OutDataTypeStr=Bus: I_ModArg
  wires:
  In1/1 -> " "/1
  In2/1 -> "  "/1
  In3/1 -> "  1"/1
  In4/1 -> " 1"/1
  In6/1 -> "  3"/1
  In5/1 -> "  2"/1
  "  3"/1 -> Bus Creator2/5  "Ic_mod"
  Gain4/1 -> Bus Creator2/4  "Ib_arg"
  Bus Creator2/1 -> Out2/1  "I_ModArg"
  Gain3/1 -> Bus Creator2/2  "Ia_arg"
  "  1"/1 -> Bus Creator1/5  "Vc_mod"
  " "/1 -> Bus Creator1/1  "Va_mod"
  Gain5/1 -> Bus Creator2/6  "Ic_arg"
  Gain/1 -> Bus Creator1/2  "Va_arg"
  "  2"/2 -> Gain4/1
  "  "/1 -> Bus Creator1/3  "Vb_mod"
  "  "/2 -> Gain1/1
  Bus Creator1/1 -> Out1/1  "V_ModArg"
  Gain1/1 -> Bus Creator1/4  "Vb_arg"
  "  1"/2 -> Gain2/1
  Gain2/1 -> Bus Creator1/6  "Vc_arg"
  " 1"/1 -> Bus Creator2/1  "Ia_mod"
  "  2"/1 -> Bus Creator2/3  "Ib_mod"
  " 1"/2 -> Gain3/1
  "  3"/2 -> Gain5/1
  " "/2 -> Gain/1

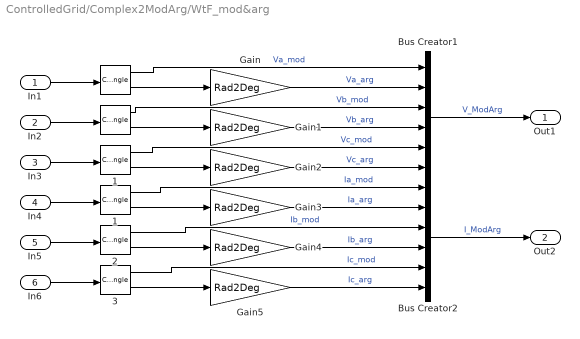
== system ControlledGrid/Complex2ModArg/WtF_mod&arg ==
  In1 : Inport
  In2 : Inport  Port=2
  In3 : Inport  Port=3
  In4 : Inport  Port=4
  In5 : Inport  Port=5
  In6 : Inport  Port=6
  " " : ComplexToMagnitudeAngle
    {,1..3} (4 alike) : ComplexToMagnitudeAngle
  " 1" : ComplexToMagnitudeAngle
  Bus Creator1 : BusCreator  Inputs=6
  Bus Creator2 : BusCreator  Inputs=6
  Gain{,1..5} (6 alike) : Gain  Gain=Rad2Deg
  Out1 : Outport  OutDataTypeStr=Bus: V_ModArg
  Out2 : Outport  Port=2  OutDataTypeStr=Bus: I_ModArg
  wires:
  In1/1 -> " "/1
  In2/1 -> "  "/1
  In3/1 -> "  1"/1
  In4/1 -> " 1"/1
  In6/1 -> "  3"/1
  In5/1 -> "  2"/1
  "  3"/1 -> Bus Creator2/5  "Ic_mod"
  Gain4/1 -> Bus Creator2/4  "Ib_arg"
  Bus Creator2/1 -> Out2/1  "I_ModArg"
  Gain3/1 -> Bus Creator2/2  "Ia_arg"
  "  1"/1 -> Bus Creator1/5  "Vc_mod"
  " "/1 -> Bus Creator1/1  "Va_mod"
  Gain5/1 -> Bus Creator2/6  "Ic_arg"
  Gain/1 -> Bus Creator1/2  "Va_arg"
  "  2"/2 -> Gain4/1
  "  "/1 -> Bus Creator1/3  "Vb_mod"
  "  "/2 -> Gain1/1
  Bus Creator1/1 -> Out1/1  "V_ModArg"
  Gain1/1 -> Bus Creator1/4  "Vb_arg"
  "  1"/2 -> Gain2/1
  Gain2/1 -> Bus Creator1/6  "Vc_arg"
  " 1"/1 -> Bus Creator2/1  "Ia_mod"
  "  2"/1 -> Bus Creator2/3  "Ib_mod"
  " 1"/2 -> Gain3/1
  "  3"/2 -> Gain5/1
  " "/2 -> Gain/1

== system ControlledGrid/ConectionNet/Subsystem ==
  In1 : Inport
  Complex to Real-Imag : ComplexToRealImag
  Gain : Gain  Gain=sqrt(3)/sqrt(2)
  Scope2 : Scope  NumInputPorts=2
  Selector : Selector  InputPortWidth=3  IndexOptions=Index vector (dialog)  Indices=[1]  OutputSizes=1
  Selector1 : Selector  InputPortWidth=3  IndexOptions=Index vector (dialog)  Indices=[1]  OutputSizes=1
  wires:
  Complex to Real-Imag/2 -> Selector1/1
  Gain/1 -> Complex to Real-Imag/1
  In1/1 -> Gain/1
  Selector/1 -> Scope2/1
  Selector1/1 -> Scope2/2
  Complex to Real-Imag/1 -> Selector/1

== system ControlledGrid/ConectionNet/Subsystem1 ==
  In1 : Inport
  Complex to Real-Imag : ComplexToRealImag
  Gain : Gain  Gain=sqrt(3)/sqrt(2)
  Scope2 : Scope  NumInputPorts=2
  Selector : Selector  InputPortWidth=3  IndexOptions=Index vector (dialog)  Indices=[1]  OutputSizes=1
  Selector1 : Selector  InputPortWidth=3  IndexOptions=Index vector (dialog)  Indices=[1]  OutputSizes=1
  wires:
  Complex to Real-Imag/1 -> Selector/1
  Selector1/1 -> Scope2/2
  Selector/1 -> Scope2/1
  In1/1 -> Gain/1
  Gain/1 -> Complex to Real-Imag/1
  Complex to Real-Imag/2 -> Selector1/1

== system ControlledGrid/ConectionNet/Subsystem2 ==
  In1 : Inport
  Complex to Real-Imag : ComplexToRealImag
  Gain : Gain  Gain=sqrt(3)/sqrt(2)
  Scope2 : Scope  NumInputPorts=2
  Selector : Selector  InputPortWidth=3  IndexOptions=Index vector (dialog)  Indices=[1]  OutputSizes=1
  Selector1 : Selector  InputPortWidth=3  IndexOptions=Index vector (dialog)  Indices=[1]  OutputSizes=1
  wires:
  Complex to Real-Imag/2 -> Selector1/1
  Gain/1 -> Complex to Real-Imag/1
  In1/1 -> Gain/1
  Selector/1 -> Scope2/1
  Selector1/1 -> Scope2/2
  Complex to Real-Imag/1 -> Selector/1

== system ControlledGrid/ConectionNet/Subsystem3 ==
  In1 : Inport
  Complex to Real-Imag : ComplexToRealImag
  Gain : Gain  Gain=sqrt(3)/sqrt(2)
  Scope2 : Scope  NumInputPorts=2
  Selector : Selector  InputPortWidth=3  IndexOptions=Index vector (dialog)  Indices=[1]  OutputSizes=1
  Selector1 : Selector  InputPortWidth=3  IndexOptions=Index vector (dialog)  Indices=[1]  OutputSizes=1
  wires:
  Complex to Real-Imag/1 -> Selector/1
  Selector1/1 -> Scope2/2
  Selector/1 -> Scope2/1
  In1/1 -> Gain/1
  Gain/1 -> Complex to Real-Imag/1
  Complex to Real-Imag/2 -> Selector1/1

== system ControlledGrid/ConectionNet/Subsystem4 ==
  In1 : Inport
  Complex to Real-Imag : ComplexToRealImag
  Gain : Gain  Gain=1/sqrt(2)
  Scope2 : Scope  NumInputPorts=2
  Selector : Selector  InputPortWidth=3  IndexOptions=Index vector (dialog)  Indices=[1]  OutputSizes=1
  Selector1 : Selector  InputPortWidth=3  IndexOptions=Index vector (dialog)  Indices=[1]  OutputSizes=1
  wires:
  Gain/1 -> Complex to Real-Imag/1
  Complex to Real-Imag/2 -> Selector1/1
  Selector/1 -> Scope2/1
  Selector1/1 -> Scope2/2
  Complex to Real-Imag/1 -> Selector/1
  In1/1 -> Gain/1

== system ControlledGrid/ConectionNet/Subsystem5 ==
  In1 : Inport
  Complex to Real-Imag : ComplexToRealImag
  Gain : Gain  Gain=1/sqrt(2)
  Scope2 : Scope  NumInputPorts=2
  Selector : Selector  InputPortWidth=3  IndexOptions=Index vector (dialog)  Indices=[1]  OutputSizes=1
  Selector1 : Selector  InputPortWidth=3  IndexOptions=Index vector (dialog)  Indices=[1]  OutputSizes=1
  wires:
  In1/1 -> Gain/1
  Complex to Real-Imag/1 -> Selector/1
  Selector1/1 -> Scope2/2
  Selector/1 -> Scope2/1
  Complex to Real-Imag/2 -> Selector1/1
  Gain/1 -> Complex to Real-Imag/1

== system ControlledGrid/ConectionNet/Subsystem6 ==
  In1 : Inport
  Complex to Real-Imag : ComplexToRealImag
  Gain : Gain  Gain=1/sqrt(2)
  Scope2 : Scope  NumInputPorts=2
  Selector : Selector  InputPortWidth=3  IndexOptions=Index vector (dialog)  Indices=[1]  OutputSizes=1
  Selector1 : Selector  InputPortWidth=3  IndexOptions=Index vector (dialog)  Indices=[1]  OutputSizes=1
  wires:
  Gain/1 -> Complex to Real-Imag/1
  Complex to Real-Imag/2 -> Selector1/1
  Selector/1 -> Scope2/1
  Selector1/1 -> Scope2/2
  Complex to Real-Imag/1 -> Selector/1
  In1/1 -> Gain/1

== system ControlledGrid/ConectionNet/Subsystem7 ==
  In1 : Inport
  Complex to Real-Imag : ComplexToRealImag
  Gain : Gain  Gain=1/sqrt(2)
  Scope2 : Scope  NumInputPorts=2
  Selector : Selector  InputPortWidth=3  IndexOptions=Index vector (dialog)  Indices=[1]  OutputSizes=1
  Selector1 : Selector  InputPortWidth=3  IndexOptions=Index vector (dialog)  Indices=[1]  OutputSizes=1
  wires:
  In1/1 -> Gain/1
  Complex to Real-Imag/1 -> Selector/1
  Selector1/1 -> Scope2/2
  Selector/1 -> Scope2/1
  Complex to Real-Imag/2 -> Selector1/1
  Gain/1 -> Complex to Real-Imag/1

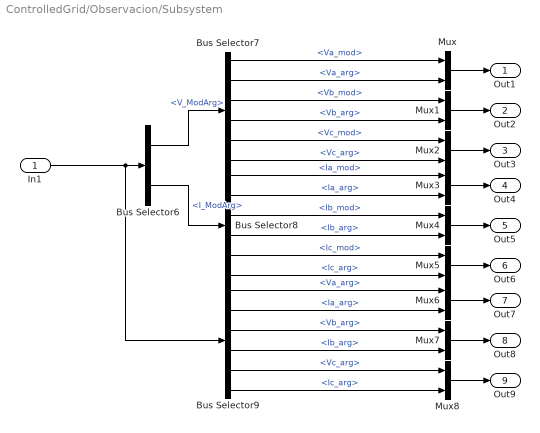
== system ControlledGrid/Observacion/Subsystem ==
  In1 : Inport  OutDataTypeStr=Bus: MV_ModArg
  Bus Selector6 : BusSelector  OutputSignals=V_ModArg,I_ModArg
  Bus Selector7 : BusSelector  OutputSignals=Va_mod,Va_arg,Vb_mod,Vb_arg,Vc_mod,Vc_arg
  Bus Selector8 : BusSelector  OutputSignals=Ia_mod,Ia_arg,Ib_mod,Ib_arg,Ic_mod,Ic_arg
  Bus Selector9 : BusSelector  OutputSignals=V_ModArg.Va_arg,I_ModArg.Ia_arg,V_ModArg.Vb_arg,I_ModArg.Ib_arg,V_ModArg.Vc_arg,I_ModArg.Ic_arg
  Mux{,1..8} (9 alike) : Mux  Inputs=2
  Out1 : Outport
  Out2 : Outport  Port=2
  Out3 : Outport  Port=3
  Out4 : Outport  Port=4
  Out5 : Outport  Port=5
  Out6 : Outport  Port=6
  Out7 : Outport  Port=7
  Out8 : Outport  Port=8
  Out9 : Outport  Port=9
  wires:
  Mux/1 -> Out1/1
  Bus Selector6/1 -> Bus Selector7/1  "<V_ModArg>"
  Bus Selector7/1 -> Mux/1  "<Va_mod>"
  Bus Selector9/4 -> Mux7/2  "<Ib_arg>"
  Mux6/1 -> Out7/1
  Mux7/1 -> Out8/1
  Bus Selector9/3 -> Mux7/1  "<Vb_arg>"
  Bus Selector9/6 -> Mux8/2  "<Ic_arg>"
  Bus Selector9/1 -> Mux6/1  "<Va_arg>"
  Bus Selector9/2 -> Mux6/2  "<Ia_arg>"
  Mux8/1 -> Out9/1
  Bus Selector9/5 -> Mux8/1  "<Vc_arg>"
  Bus Selector7/3 -> Mux1/1  "<Vb_mod>"
  Bus Selector7/5 -> Mux2/1  "<Vc_mod>"
  Bus Selector7/6 -> Mux2/2  "<Vc_arg>"
  Mux2/1 -> Out3/1
  Mux1/1 -> Out2/1
  Bus Selector7/2 -> Mux/2  "<Va_arg>"
  Bus Selector8/6 -> Mux5/2  "<Ic_arg>"
  Bus Selector8/4 -> Mux4/2  "<Ib_arg>"
  Bus Selector8/1 -> Mux3/1  "<Ia_mod>"
  Mux3/1 -> Out4/1
  Bus Selector8/5 -> Mux5/1  "<Ic_mod>"
  Mux4/1 -> Out5/1
  Bus Selector8/3 -> Mux4/1  "<Ib_mod>"
  Bus Selector8/2 -> Mux3/2  "<Ia_arg>"
  Mux5/1 -> Out6/1
  Bus Selector6/2 -> Bus Selector8/1  "<I_ModArg>"
  Bus Selector7/4 -> Mux1/2  "<Vb_arg>"
  In1/1 -> Bus Selector9/1, Bus Selector6/1

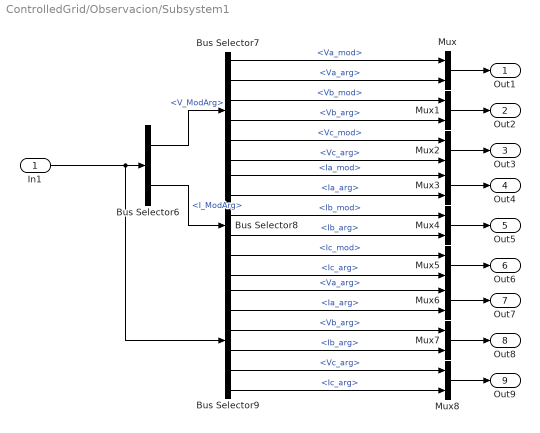
== system ControlledGrid/Observacion/Subsystem1 ==
  In1 : Inport  OutDataTypeStr=Bus: HV_ModArg
  Bus Selector6 : BusSelector  OutputSignals=V_ModArg,I_ModArg
  Bus Selector7 : BusSelector  OutputSignals=Va_mod,Va_arg,Vb_mod,Vb_arg,Vc_mod,Vc_arg
  Bus Selector8 : BusSelector  OutputSignals=Ia_mod,Ia_arg,Ib_mod,Ib_arg,Ic_mod,Ic_arg
  Bus Selector9 : BusSelector  OutputSignals=V_ModArg.Va_arg,I_ModArg.Ia_arg,V_ModArg.Vb_arg,I_ModArg.Ib_arg,V_ModArg.Vc_arg,I_ModArg.Ic_arg
  Mux{,1..8} (9 alike) : Mux  Inputs=2
  Out1 : Outport
  Out2 : Outport  Port=2
  Out3 : Outport  Port=3
  Out4 : Outport  Port=4
  Out5 : Outport  Port=5
  Out6 : Outport  Port=6
  Out7 : Outport  Port=7
  Out8 : Outport  Port=8
  Out9 : Outport  Port=9
  wires:
  In1/1 -> Bus Selector6/1, Bus Selector9/1
  Bus Selector7/4 -> Mux1/2  "<Vb_arg>"
  Bus Selector6/2 -> Bus Selector8/1  "<I_ModArg>"
  Mux5/1 -> Out6/1
  Bus Selector8/2 -> Mux3/2  "<Ia_arg>"
  Bus Selector8/3 -> Mux4/1  "<Ib_mod>"
  Mux4/1 -> Out5/1
  Bus Selector8/5 -> Mux5/1  "<Ic_mod>"
  Mux3/1 -> Out4/1
  Bus Selector8/1 -> Mux3/1  "<Ia_mod>"
  Bus Selector8/4 -> Mux4/2  "<Ib_arg>"
  Bus Selector8/6 -> Mux5/2  "<Ic_arg>"
  Bus Selector7/2 -> Mux/2  "<Va_arg>"
  Mux1/1 -> Out2/1
  Mux2/1 -> Out3/1
  Bus Selector7/6 -> Mux2/2  "<Vc_arg>"
  Bus Selector7/5 -> Mux2/1  "<Vc_mod>"
  Bus Selector7/3 -> Mux1/1  "<Vb_mod>"
  Bus Selector9/5 -> Mux8/1  "<Vc_arg>"
  Mux8/1 -> Out9/1
  Bus Selector9/2 -> Mux6/2  "<Ia_arg>"
  Bus Selector9/1 -> Mux6/1  "<Va_arg>"
  Bus Selector9/6 -> Mux8/2  "<Ic_arg>"
  Bus Selector9/3 -> Mux7/1  "<Vb_arg>"
  Mux7/1 -> Out8/1
  Mux6/1 -> Out7/1
  Bus Selector9/4 -> Mux7/2  "<Ib_arg>"
  Bus Selector7/1 -> Mux/1  "<Va_mod>"
  Bus Selector6/1 -> Bus Selector7/1  "<V_ModArg>"
  Mux/1 -> Out1/1

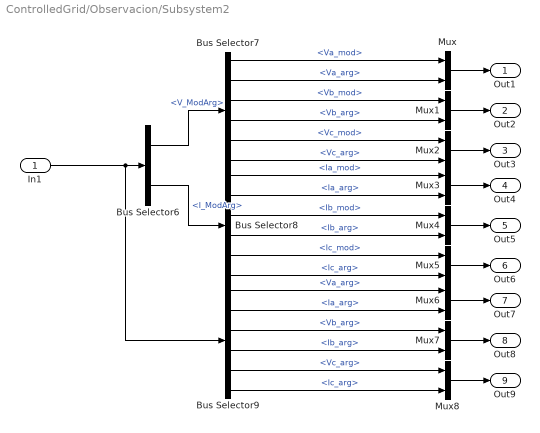
== system ControlledGrid/Observacion/Subsystem2 ==
  In1 : Inport  OutDataTypeStr=Bus: WtF_ModArg
  Bus Selector6 : BusSelector  OutputSignals=V_ModArg,I_ModArg
  Bus Selector7 : BusSelector  OutputSignals=Va_mod,Va_arg,Vb_mod,Vb_arg,Vc_mod,Vc_arg
  Bus Selector8 : BusSelector  OutputSignals=Ia_mod,Ia_arg,Ib_mod,Ib_arg,Ic_mod,Ic_arg
  Bus Selector9 : BusSelector  OutputSignals=V_ModArg.Va_arg,I_ModArg.Ia_arg,V_ModArg.Vb_arg,I_ModArg.Ib_arg,V_ModArg.Vc_arg,I_ModArg.Ic_arg
  Mux{,1..8} (9 alike) : Mux  Inputs=2
  Out1 : Outport
  Out2 : Outport  Port=2
  Out3 : Outport  Port=3
  Out4 : Outport  Port=4
  Out5 : Outport  Port=5
  Out6 : Outport  Port=6
  Out7 : Outport  Port=7
  Out8 : Outport  Port=8
  Out9 : Outport  Port=9
  wires:
  Mux/1 -> Out1/1
  Bus Selector6/1 -> Bus Selector7/1  "<V_ModArg>"
  Bus Selector7/1 -> Mux/1  "<Va_mod>"
  Bus Selector9/4 -> Mux7/2  "<Ib_arg>"
  Mux6/1 -> Out7/1
  Mux7/1 -> Out8/1
  Bus Selector9/3 -> Mux7/1  "<Vb_arg>"
  Bus Selector9/6 -> Mux8/2  "<Ic_arg>"
  Bus Selector9/1 -> Mux6/1  "<Va_arg>"
  Bus Selector9/2 -> Mux6/2  "<Ia_arg>"
  Mux8/1 -> Out9/1
  Bus Selector9/5 -> Mux8/1  "<Vc_arg>"
  Bus Selector7/3 -> Mux1/1  "<Vb_mod>"
  Bus Selector7/5 -> Mux2/1  "<Vc_mod>"
  Bus Selector7/6 -> Mux2/2  "<Vc_arg>"
  Mux2/1 -> Out3/1
  Mux1/1 -> Out2/1
  Bus Selector7/2 -> Mux/2  "<Va_arg>"
  Bus Selector8/6 -> Mux5/2  "<Ic_arg>"
  Bus Selector8/4 -> Mux4/2  "<Ib_arg>"
  Bus Selector8/1 -> Mux3/1  "<Ia_mod>"
  Mux3/1 -> Out4/1
  Bus Selector8/5 -> Mux5/1  "<Ic_mod>"
  Mux4/1 -> Out5/1
  Bus Selector8/3 -> Mux4/1  "<Ib_mod>"
  Bus Selector8/2 -> Mux3/2  "<Ia_arg>"
  Mux5/1 -> Out6/1
  Bus Selector6/2 -> Bus Selector8/1  "<I_ModArg>"
  Bus Selector7/4 -> Mux1/2  "<Vb_arg>"
  In1/1 -> Bus Selector9/1, Bus Selector6/1
